simulink model "fuel_tank_test"  (R2025a)
settings: Solver=daessc  StartTime=0.0  StopTime=1000  RelTol=1e-3
libraries: fl_lib x2, nesl_utility x1
settings Model: Creator=MW  LastModifiedBy=MW

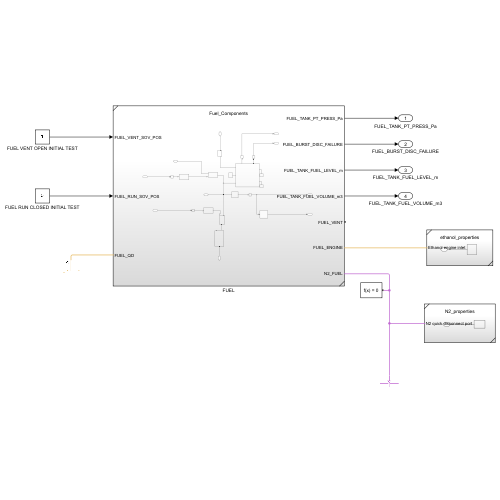
[thumbnail: Simulink's stored preview of the top-level diagram]
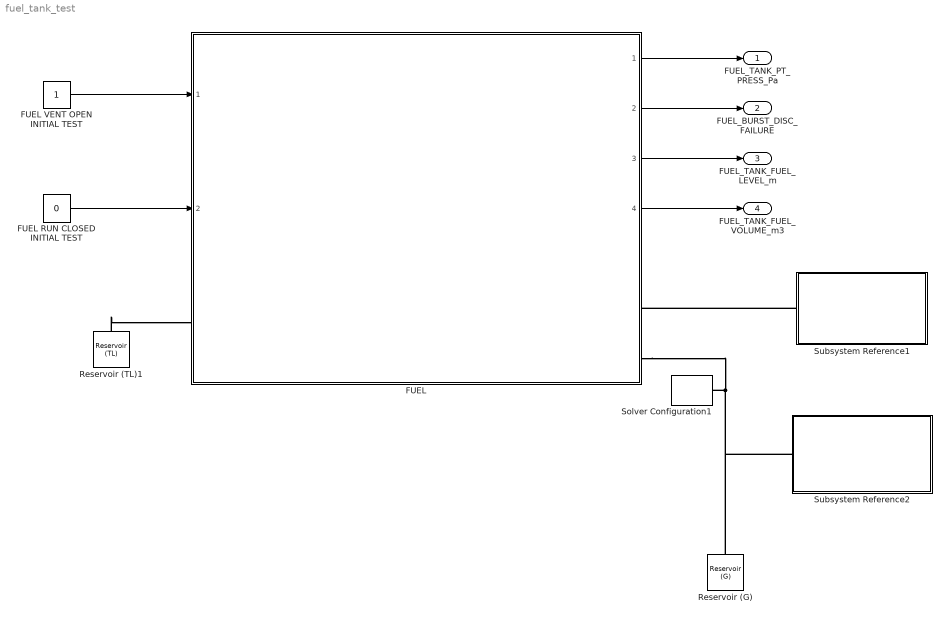
== system fuel_tank_test ==
  FUEL : Subsystem  ReferencedSubsystem=Fuel_Components
  FUEL RUN CLOSED INITIAL TEST : Constant  Value=0
  FUEL VENT OPEN INITIAL TEST : Constant
  Reservoir (G) : fl_lib/Gas/Elements/Reservoir (G)  pressure_spec=foundation.enum.pressure_spec.specified  reservoir_pressure=0.101325 MPa  reservoir_temperature=293.15 K  area_A=0.01 m^2
  Reservoir (TL)1 : fl_lib/Thermal Liquid/Elements/Reservoir (TL)  pressure_spec=foundation.enum.pressure_spec.atmospheric  reservoir_pressure=0.101325 MPa  reservoir_temperature=293.15 K  area=0.01 m^2
  Solver Configuration1 : nesl_utility/Solver Configuration  PhysicalDomain=network_engine_domain  SubClassName=solver  LeftPortType=input  RightPortType=generic  Tones=[]  Harmonics=[]  SimulateNoise=off  Profile=off  UseLocalSampling=off  EnableSwitchedLinearOptims=on  FrequencyDomain=off  UseCCode=off  RelTol=0.001  AbsTol=0.001  MinStep=1e-09  ToWorkspace=off  RevertToSquareIcSolve=off  NumHomotopyIterations=100  PhasorMode=off  PhasorModeNumHarmonics=1  ConsistencySolver=NEWTON_XTOL_AFTER_FTOL  IndexReductionMethod=DerivativeReplacement  DoDC=off  ResidualTolerance=1e-09  ConsistencyTolSource=GLOBAL  ConsistencyAbsTol=0.001  ConsistencyRelTol=0.001  ConsistencyTolFactor=0.001  UseLocalSolver=off  LocalSolverChoice=NE_BACKWARD_EULER_ADVANCER  ResolveIndetEquations=on  FunctionEvalNumThread=1  LocalSolverSampleTime=0.001  DoFixedCost=off  MaxNonlinIter=3  MaxModeIter=2  ComputeImpulses=off  ImpulseIterations=2  LinearAlgebra=auto  LinearAlgebraNumThread=0  EquationFormulation=NE_TIME_EF  DelaysMemoryBudget=1024  AutomaticFiltering=on  FilteringTimeConstant=0.001  PartitionStorageMethod=AS_NEEDED  PartitionMemoryBudget=1024  PartitionMethod=ROBUST  MultibodyUseLocalSolver=off  MultibodyLocalSolverChoice=ODE1  MultibodyLocalSolverSampleTime=0.001
  Subsystem Reference1 : Subsystem  ReferencedSubsystem=ethanol_properties
  Subsystem Reference2 : Subsystem  ReferencedSubsystem=N2_properties
  FUEL_TANK_PT_PRESS_Pa : Outport
  FUEL_BURST_DISC_FAILURE : Outport  Port=2
  FUEL_TANK_FUEL_LEVEL_m : Outport  Port=3
  FUEL_TANK_FUEL_VOLUME_m3 : Outport  Port=4
  wires:
  FUEL VENT OPEN INITIAL TEST/1 -> FUEL/1
  FUEL RUN CLOSED INITIAL TEST/1 -> FUEL/2
  FUEL/1 -> FUEL_TANK_PT_PRESS_Pa/1
  FUEL/2 -> FUEL_BURST_DISC_FAILURE/1
  FUEL/3 -> FUEL_TANK_FUEL_LEVEL_m/1
  FUEL/4 -> FUEL_TANK_FUEL_VOLUME_m3/1
  connections:
  FUEL/RConn3 -- Reservoir (G)/LConn1 -- Subsystem Reference2/LConn1 -- Solver Configuration1/RConn1
  Subsystem Reference1/LConn1 -- FUEL/RConn2
  Reservoir (TL)1/LConn1 -- FUEL/LConn1
